simulink model "dual500MHzPFB"  (Simulink 6.2)
settings: Solver=ode45  StartTime=0.0  StopTime=10000  RelTol=1e-3
libraries: xbsIndex_r3 x2070, casper_library x180, xps_library x12, gtkWave x5, gavrt_library x1
(part 15 of 20)

== system dual500MHzPFB/cfgspec/FFT_Subsystem/fft_wideband_real1/fft_biplex_real_4x0/biplex_core/fft_stage_5 ==
  in1 : Inport  Port=1  LatchInput=off
  in2 : Inport  Port=2  LatchInput=off
  of_in : Inport  Port=3  LatchInput=off
  sync : Inport  Port=4  LatchInput=off
  shift : Inport  Port=5  LatchInput=off
  Counter : xbsIndex_r3/Counter  cnt_type=Free Running  n_bits=FFTSize-FFTStage+1  bin_pt=0  arith_type=Unsigned  start_count=0  cnt_to=Inf  cnt_by_val=1  operation=Up  explicit_period=off  period=1  load_pin=off  rst=on  en=off  dbl_ovrd=off  show_param=off  use_rpm=off  gen_core=on
      settings: xl_area=[0, 0, 0, 0, 0, 0, 0]
  Delay : xbsIndex_r3/Delay  latency=1  reg_retiming=off  explicit_period=off  period=1  en=off  accept_only_valid=off  init_zero=on  dbl_ovrd=off  show_param=off
      settings: xl_area=[0, 0, 0, 0, 0, 0, 0]
  Logical1 : xbsIndex_r3/Logical  logical_function=OR  inputs=2  precision=Full  arith_type=Unsigned  n_bits=8  bin_pt=2  align_bp=on  latency=1  explicit_period=on  period=1  en=off  dbl_ovrd=off  show_param=off
      settings: xl_area=[0, 0, 0, 0, 0, 0, 0]
  Mux : xbsIndex_r3/Mux  inputs=2  precision=Full  arith_type="Signed  (2's comp)"  n_bits=8  bin_pt=2  quantization=Truncate  overflow=Wrap  latency=1  explicit_period=off  period=1  en=off  dbl_ovrd=off  show_param=off  mux_type=off  use_rpm=off  gen_core=on
      settings: xl_area=[0, 0, 0, 0, 0, 0, 0]
  Mux1 : xbsIndex_r3/Mux  inputs=2  precision=Full  arith_type="Signed  (2's comp)"  n_bits=8  bin_pt=2  quantization=Truncate  overflow=Wrap  latency=1  explicit_period=off  period=1  en=off  dbl_ovrd=off  show_param=off  mux_type=off  use_rpm=off  gen_core=on
      settings: xl_area=[0, 0, 0, 0, 0, 0, 0]
  Slice : xbsIndex_r3/Slice  Orientation=up  mode=Lower Bit Location + Width  nbits=1  bit1=-(FFTStage - 1)  base1=MSB of Input  bit0=FFTStage - 1  base0=LSB of Input  boolean_output=on  explicit_period=off  period=1  dbl_ovrd=off
  Slice1 : xbsIndex_r3/Slice  mode=Upper Bit Location + Width  nbits=1  bit1=0  base1=MSB of Input  bit0=0  base0=LSB of Input  boolean_output=off  explicit_period=off  period=1  dbl_ovrd=off
  butterfly_direct : Subsystem  AncestorBlock=casper_library/FFTs/butterfly_direct  mask(butterfly_direct){FFTSize=8, Coeffs=[0 1 2 3 4 5 6 7 8 9 10 11 12 13 14 15], StepPeriod=3, BitWidth=18, add_latency=3, mult_latency=3, bram_latency=2, use_bram=0, quantization=Truncate, overflow=Wrap}
      mask prompts: FFTSize "Size of FFT: (2^?)"; Coeffs "Coefficients: (0 to 2^(FFTSize-1)-1)"; StepPeriod "Coefficient Step Period: (2^?)"; BitWidth "Output Bitwidth:"; add_latency "Add Latency"; mult_latency "Mult Latency"; bram_latency "BRAM Latency"; use_bram "Store Coefficients in BRAM"; quantization "Quantization Behavior"; overflow "Overflow Behavior"
      mask init: same as dual500MHzPFB/cfgspec/FFT_Subsystem/fft_wideband_real/fft_direct/butterfly1_0
      settings: AttributesFormatString=|
      | FFTSize=8, Coeffs=[0   1   2   3   4   5   6   7   8   9  10  11  12  13  14  15],
      |  StepPeriod=3, BitWidth=18
      mask StyleString: edit,edit,edit,edit,edit,edit,edit,edit,popup(Truncate|Round  (unbiased: +/- Inf)|Round  (unbiased: Even Values)),popup(Wrap|Saturate|Error)
  delay_b : Subsystem  BlockChoice=delay_slr
      link override delay_bram: bram_latency=bram_latency  DelayLen=2^(FFTSize-FFTStage)
      link override delay_slr: DelayLen=2^(FFTSize-FFTStage)
      settings: AttributesFormatString=%<BlockChoice>  TemplateBlock=casper_library/Delays/delay  MemberBlocks=delay_bram,delay_slr
  delay_f : Subsystem  BlockChoice=delay_slr
      link override delay_bram: bram_latency=bram_latency  DelayLen=2^(FFTSize-FFTStage)
      link override delay_slr: DelayLen=2^(FFTSize-FFTStage)
      settings: AttributesFormatString=%<BlockChoice>  TemplateBlock=casper_library/Delays/delay  MemberBlocks=delay_bram,delay_slr
  sync_delay : casper_library/Delays/sync_delay  DelayLen=2^(FFTSize - FFTStage)
      link override Constant: equ=P=C
      link override Constant1: equ=P=C
      link override Constant2: equ=P=C
      link override Constant3: equ=P=C
  out1 : Outport
  out2 : Outport  Port=2
  of : Outport  Port=3
  sync_out : Outport  Port=4
  wires:
  butterfly_direct/4(sync_out) -> sync_out/1
  butterfly_direct/1(a+bw) -> out1/1
  butterfly_direct/2(a-bw) -> out2/1
  butterfly_direct/3(of) -> Logical1/1
  Slice/1 -> butterfly_direct/4(shift)
  sync_delay/1 -> butterfly_direct/3(sync)
  delay_b/1(Out1) -> butterfly_direct/1(a)
  in2/1 -> delay_f/1(In1)
  Slice1/1 -> Mux1/1, Mux/1
  in1/1 -> Mux1/2, Mux/3
  delay_f/1(Out1) -> Mux/2, Mux1/3
  Mux1/1 -> delay_b/1(In1)
  Mux/1 -> butterfly_direct/2(b)
  Counter/1 -> Slice1/1
  sync/1 -> Delay/1, Counter/1
  Delay/1 -> sync_delay/1
  Logical1/1 -> of/1
  of_in/1 -> Logical1/2
  shift/1 -> Slice/1

== system dual500MHzPFB/cfgspec/FFT_Subsystem/fft_wideband_real1/fft_biplex_real_4x0/biplex_core/fft_stage_6 ==
  in1 : Inport  Port=1  LatchInput=off
  in2 : Inport  Port=2  LatchInput=off
  of_in : Inport  Port=3  LatchInput=off
  sync : Inport  Port=4  LatchInput=off
  shift : Inport  Port=5  LatchInput=off
  Counter : xbsIndex_r3/Counter  cnt_type=Free Running  n_bits=FFTSize-FFTStage+1  bin_pt=0  arith_type=Unsigned  start_count=0  cnt_to=Inf  cnt_by_val=1  operation=Up  explicit_period=off  period=1  load_pin=off  rst=on  en=off  dbl_ovrd=off  show_param=off  use_rpm=off  gen_core=on
      settings: xl_area=[0, 0, 0, 0, 0, 0, 0]
  Delay : xbsIndex_r3/Delay  latency=1  reg_retiming=off  explicit_period=off  period=1  en=off  accept_only_valid=off  init_zero=on  dbl_ovrd=off  show_param=off
      settings: xl_area=[0, 0, 0, 0, 0, 0, 0]
  Logical1 : xbsIndex_r3/Logical  logical_function=OR  inputs=2  precision=Full  arith_type=Unsigned  n_bits=8  bin_pt=2  align_bp=on  latency=1  explicit_period=on  period=1  en=off  dbl_ovrd=off  show_param=off
      settings: xl_area=[0, 0, 0, 0, 0, 0, 0]
  Mux : xbsIndex_r3/Mux  inputs=2  precision=Full  arith_type="Signed  (2's comp)"  n_bits=8  bin_pt=2  quantization=Truncate  overflow=Wrap  latency=1  explicit_period=off  period=1  en=off  dbl_ovrd=off  show_param=off  mux_type=off  use_rpm=off  gen_core=on
      settings: xl_area=[0, 0, 0, 0, 0, 0, 0]
  Mux1 : xbsIndex_r3/Mux  inputs=2  precision=Full  arith_type="Signed  (2's comp)"  n_bits=8  bin_pt=2  quantization=Truncate  overflow=Wrap  latency=1  explicit_period=off  period=1  en=off  dbl_ovrd=off  show_param=off  mux_type=off  use_rpm=off  gen_core=on
      settings: xl_area=[0, 0, 0, 0, 0, 0, 0]
  Slice : xbsIndex_r3/Slice  Orientation=up  mode=Lower Bit Location + Width  nbits=1  bit1=-(FFTStage - 1)  base1=MSB of Input  bit0=FFTStage - 1  base0=LSB of Input  boolean_output=on  explicit_period=off  period=1  dbl_ovrd=off
  Slice1 : xbsIndex_r3/Slice  mode=Upper Bit Location + Width  nbits=1  bit1=0  base1=MSB of Input  bit0=0  base0=LSB of Input  boolean_output=off  explicit_period=off  period=1  dbl_ovrd=off
  butterfly_direct : Subsystem  AncestorBlock=casper_library/FFTs/butterfly_direct  mask(butterfly_direct){FFTSize=8, Coeffs=[0 1 2 3 4 5 6 7 8 9 10 11 12 13 14 15 16 17 18 19 20 21 22 23 24 25 26 27 28 29 30 31], StepPeriod=2, BitWidth=18, add_latency=3, mult_latency=3, bram_latency=2, use_bram=0, quantization=Truncate, overflow=Wrap}
      mask prompts: FFTSize "Size of FFT: (2^?)"; Coeffs "Coefficients: (0 to 2^(FFTSize-1)-1)"; StepPeriod "Coefficient Step Period: (2^?)"; BitWidth "Output Bitwidth:"; add_latency "Add Latency"; mult_latency "Mult Latency"; bram_latency "BRAM Latency"; use_bram "Store Coefficients in BRAM"; quantization "Quantization Behavior"; overflow "Overflow Behavior"
      mask init: same as dual500MHzPFB/cfgspec/FFT_Subsystem/fft_wideband_real/fft_direct/butterfly1_0
      settings: AttributesFormatString=|
      | FFTSize=8, Coeffs=[0   1   2   3   4   5   6   7   8   9  10  11  12  13  14  15  16  17  18  19  20  21  22  23  24  25  26  27  28  29  30  31],
      |  StepPeriod=2, BitWidth=18
      mask StyleString: edit,edit,edit,edit,edit,edit,edit,edit,popup(Truncate|Round  (unbiased: +/- Inf)|Round  (unbiased: Even Values)),popup(Wrap|Saturate|Error)
  delay_b : Subsystem  BlockChoice=delay_slr
      link override delay_bram: bram_latency=bram_latency  DelayLen=2^(FFTSize-FFTStage)
      link override delay_slr: DelayLen=2^(FFTSize-FFTStage)
      settings: AttributesFormatString=%<BlockChoice>  TemplateBlock=casper_library/Delays/delay  MemberBlocks=delay_bram,delay_slr
  delay_f : Subsystem  BlockChoice=delay_slr
      link override delay_bram: bram_latency=bram_latency  DelayLen=2^(FFTSize-FFTStage)
      link override delay_slr: DelayLen=2^(FFTSize-FFTStage)
      settings: AttributesFormatString=%<BlockChoice>  TemplateBlock=casper_library/Delays/delay  MemberBlocks=delay_bram,delay_slr
  sync_delay : casper_library/Delays/sync_delay  DelayLen=2^(FFTSize - FFTStage)
      link override Constant: equ=P=C
      link override Constant1: equ=P=C
      link override Constant2: equ=P=C
      link override Constant3: equ=P=C
  out1 : Outport
  out2 : Outport  Port=2
  of : Outport  Port=3
  sync_out : Outport  Port=4
  wires:
  butterfly_direct/4(sync_out) -> sync_out/1
  butterfly_direct/1(a+bw) -> out1/1
  butterfly_direct/2(a-bw) -> out2/1
  butterfly_direct/3(of) -> Logical1/1
  Slice/1 -> butterfly_direct/4(shift)
  sync_delay/1 -> butterfly_direct/3(sync)
  delay_b/1(Out1) -> butterfly_direct/1(a)
  in2/1 -> delay_f/1(In1)
  Slice1/1 -> Mux1/1, Mux/1
  in1/1 -> Mux1/2, Mux/3
  delay_f/1(Out1) -> Mux/2, Mux1/3
  Mux1/1 -> delay_b/1(In1)
  Mux/1 -> butterfly_direct/2(b)
  Counter/1 -> Slice1/1
  sync/1 -> Delay/1, Counter/1
  Delay/1 -> sync_delay/1
  Logical1/1 -> of/1
  of_in/1 -> Logical1/2
  shift/1 -> Slice/1

== system dual500MHzPFB/cfgspec/FFT_Subsystem/fft_wideband_real1/fft_biplex_real_4x0/biplex_core/fft_stage_7 ==
  in1 : Inport  Port=1  LatchInput=off
  in2 : Inport  Port=2  LatchInput=off
  of_in : Inport  Port=3  LatchInput=off
  sync : Inport  Port=4  LatchInput=off
  shift : Inport  Port=5  LatchInput=off
  Counter : xbsIndex_r3/Counter  cnt_type=Free Running  n_bits=FFTSize-FFTStage+1  bin_pt=0  arith_type=Unsigned  start_count=0  cnt_to=Inf  cnt_by_val=1  operation=Up  explicit_period=off  period=1  load_pin=off  rst=on  en=off  dbl_ovrd=off  show_param=off  use_rpm=off  gen_core=on
      settings: xl_area=[0, 0, 0, 0, 0, 0, 0]
  Delay : xbsIndex_r3/Delay  latency=1  reg_retiming=off  explicit_period=off  period=1  en=off  accept_only_valid=off  init_zero=on  dbl_ovrd=off  show_param=off
      settings: xl_area=[0, 0, 0, 0, 0, 0, 0]
  Logical1 : xbsIndex_r3/Logical  logical_function=OR  inputs=2  precision=Full  arith_type=Unsigned  n_bits=8  bin_pt=2  align_bp=on  latency=1  explicit_period=on  period=1  en=off  dbl_ovrd=off  show_param=off
      settings: xl_area=[0, 0, 0, 0, 0, 0, 0]
  Mux : xbsIndex_r3/Mux  inputs=2  precision=Full  arith_type="Signed  (2's comp)"  n_bits=8  bin_pt=2  quantization=Truncate  overflow=Wrap  latency=1  explicit_period=off  period=1  en=off  dbl_ovrd=off  show_param=off  mux_type=off  use_rpm=off  gen_core=on
      settings: xl_area=[0, 0, 0, 0, 0, 0, 0]
  Mux1 : xbsIndex_r3/Mux  inputs=2  precision=Full  arith_type="Signed  (2's comp)"  n_bits=8  bin_pt=2  quantization=Truncate  overflow=Wrap  latency=1  explicit_period=off  period=1  en=off  dbl_ovrd=off  show_param=off  mux_type=off  use_rpm=off  gen_core=on
      settings: xl_area=[0, 0, 0, 0, 0, 0, 0]
  Slice : xbsIndex_r3/Slice  Orientation=up  mode=Lower Bit Location + Width  nbits=1  bit1=-(FFTStage - 1)  base1=MSB of Input  bit0=FFTStage - 1  base0=LSB of Input  boolean_output=on  explicit_period=off  period=1  dbl_ovrd=off
  Slice1 : xbsIndex_r3/Slice  mode=Upper Bit Location + Width  nbits=1  bit1=0  base1=MSB of Input  bit0=0  base0=LSB of Input  boolean_output=off  explicit_period=off  period=1  dbl_ovrd=off
  butterfly_direct : Subsystem  AncestorBlock=casper_library/FFTs/butterfly_direct  mask(butterfly_direct){FFTSize=8, Coeffs=[0 1 2 3 4 5 6 7 8 9 10 11 12 13 14 15 16 17 18 19 20 21 22 23 24 25 26 27 28 29 30 31 32 33 34 35 36 37 38 39 40 41 42 43 44 45 46 47 48 49 50 51 52 53 54 55 56 57 58 59 60 61 62 63], StepPeriod=1, BitWidth=18, add_latency=3, mult_latency=3, bram_latency=2, use_bram=0, quantization=Truncate, overflow=Wrap}
      mask prompts: FFTSize "Size of FFT: (2^?)"; Coeffs "Coefficients: (0 to 2^(FFTSize-1)-1)"; StepPeriod "Coefficient Step Period: (2^?)"; BitWidth "Output Bitwidth:"; add_latency "Add Latency"; mult_latency "Mult Latency"; bram_latency "BRAM Latency"; use_bram "Store Coefficients in BRAM"; quantization "Quantization Behavior"; overflow "Overflow Behavior"
      mask init: same as dual500MHzPFB/cfgspec/FFT_Subsystem/fft_wideband_real/fft_direct/butterfly1_0
      settings: AttributesFormatString=|
      | FFTSize=8, Coeffs=[0   1   2   3   4   5   6   7   8   9  10  11  12  13  14  15  16  17  18  19  20  21  22  23  24  25  26  27  28  29  30  31  32  33  34  35  36  37  38  39  40  41  42  43  44  45  46  47  48  49  50  51  52  53  54  55  56  57  58  59  60  61  62  63],
      |  StepPeriod=1, BitWidth=18
      mask StyleString: edit,edit,edit,edit,edit,edit,edit,edit,popup(Truncate|Round  (unbiased: +/- Inf)|Round  (unbiased: Even Values)),popup(Wrap|Saturate|Error)
  delay_b : Subsystem  BlockChoice=delay_slr
      link override delay_bram: bram_latency=bram_latency  DelayLen=2^(FFTSize-FFTStage)
      link override delay_slr: DelayLen=2^(FFTSize-FFTStage)
      settings: AttributesFormatString=%<BlockChoice>  TemplateBlock=casper_library/Delays/delay  MemberBlocks=delay_bram,delay_slr
  delay_f : Subsystem  BlockChoice=delay_slr
      link override delay_bram: bram_latency=bram_latency  DelayLen=2^(FFTSize-FFTStage)
      link override delay_slr: DelayLen=2^(FFTSize-FFTStage)
      settings: AttributesFormatString=%<BlockChoice>  TemplateBlock=casper_library/Delays/delay  MemberBlocks=delay_bram,delay_slr
  sync_delay : casper_library/Delays/sync_delay  DelayLen=2^(FFTSize - FFTStage)
      link override Constant: equ=P=C
      link override Constant1: equ=P=C
      link override Constant2: equ=P=C
      link override Constant3: equ=P=C
  out1 : Outport
  out2 : Outport  Port=2
  of : Outport  Port=3
  sync_out : Outport  Port=4
  wires:
  butterfly_direct/4(sync_out) -> sync_out/1
  butterfly_direct/1(a+bw) -> out1/1
  butterfly_direct/2(a-bw) -> out2/1
  butterfly_direct/3(of) -> Logical1/1
  Slice/1 -> butterfly_direct/4(shift)
  sync_delay/1 -> butterfly_direct/3(sync)
  delay_b/1(Out1) -> butterfly_direct/1(a)
  in2/1 -> delay_f/1(In1)
  Slice1/1 -> Mux1/1, Mux/1
  in1/1 -> Mux1/2, Mux/3
  delay_f/1(Out1) -> Mux/2, Mux1/3
  Mux1/1 -> delay_b/1(In1)
  Mux/1 -> butterfly_direct/2(b)
  Counter/1 -> Slice1/1
  sync/1 -> Delay/1, Counter/1
  Delay/1 -> sync_delay/1
  Logical1/1 -> of/1
  of_in/1 -> Logical1/2
  shift/1 -> Slice/1

== system dual500MHzPFB/cfgspec/FFT_Subsystem/fft_wideband_real1/fft_biplex_real_4x0/biplex_core/fft_stage_8 ==
  in1 : Inport  Port=1  LatchInput=off
  in2 : Inport  Port=2  LatchInput=off
  of_in : Inport  Port=3  LatchInput=off
  sync : Inport  Port=4  LatchInput=off
  shift : Inport  Port=5  LatchInput=off
  Counter : xbsIndex_r3/Counter  cnt_type=Free Running  n_bits=FFTSize-FFTStage+1  bin_pt=0  arith_type=Unsigned  start_count=0  cnt_to=Inf  cnt_by_val=1  operation=Up  explicit_period=off  period=1  load_pin=off  rst=on  en=off  dbl_ovrd=off  show_param=off  use_rpm=off  gen_core=on
      settings: xl_area=[0, 0, 0, 0, 0, 0, 0]
  Delay : xbsIndex_r3/Delay  latency=1  reg_retiming=off  explicit_period=off  period=1  en=off  accept_only_valid=off  init_zero=on  dbl_ovrd=off  show_param=off
      settings: xl_area=[0, 0, 0, 0, 0, 0, 0]
  Logical1 : xbsIndex_r3/Logical  logical_function=OR  inputs=2  precision=Full  arith_type=Unsigned  n_bits=8  bin_pt=2  align_bp=on  latency=1  explicit_period=on  period=1  en=off  dbl_ovrd=off  show_param=off
      settings: xl_area=[0, 0, 0, 0, 0, 0, 0]
  Mux : xbsIndex_r3/Mux  inputs=2  precision=Full  arith_type="Signed  (2's comp)"  n_bits=8  bin_pt=2  quantization=Truncate  overflow=Wrap  latency=1  explicit_period=off  period=1  en=off  dbl_ovrd=off  show_param=off  mux_type=off  use_rpm=off  gen_core=on
      settings: xl_area=[0, 0, 0, 0, 0, 0, 0]
  Mux1 : xbsIndex_r3/Mux  inputs=2  precision=Full  arith_type="Signed  (2's comp)"  n_bits=8  bin_pt=2  quantization=Truncate  overflow=Wrap  latency=1  explicit_period=off  period=1  en=off  dbl_ovrd=off  show_param=off  mux_type=off  use_rpm=off  gen_core=on
      settings: xl_area=[0, 0, 0, 0, 0, 0, 0]
  Slice : xbsIndex_r3/Slice  Orientation=up  mode=Lower Bit Location + Width  nbits=1  bit1=-(FFTStage - 1)  base1=MSB of Input  bit0=FFTStage - 1  base0=LSB of Input  boolean_output=on  explicit_period=off  period=1  dbl_ovrd=off
  Slice1 : xbsIndex_r3/Slice  mode=Upper Bit Location + Width  nbits=1  bit1=0  base1=MSB of Input  bit0=0  base0=LSB of Input  boolean_output=off  explicit_period=off  period=1  dbl_ovrd=off
  butterfly_direct : Subsystem  AncestorBlock=casper_library/FFTs/butterfly_direct  mask(butterfly_direct){FFTSize=8, Coeffs=[0 1 2 3 4 5 6 7 8 9 10 11 12 13 14 15 16 17 18 19 20 21 22 23 24 25 26 27 28 29 30 31 32 33 34 35 36 37 38 39 40 41 42 43 44 45 46 47 48 49 50 51 52 53 54 55 56 57 58 59 60 61 62 63 64 65 66 67 68 69 70 71 72 73 74 75 76 77 78 79 80 81 82 83 84 85 86 87 88 89 90 91 92 93 94 95 96 97 98 99 100 101 102 103 104 105 106 107 108 109 110 111 112 113 114 115 116 117 118 119 120 121 122 123 124 125 126 127], StepPeriod=0, BitWidth=18, add_latency=3, mult_latency=3, bram_latency=2, use_bram=0, quantization=Truncate, overflow=Wrap}
      mask prompts: FFTSize "Size of FFT: (2^?)"; Coeffs "Coefficients: (0 to 2^(FFTSize-1)-1)"; StepPeriod "Coefficient Step Period: (2^?)"; BitWidth "Output Bitwidth:"; add_latency "Add Latency"; mult_latency "Mult Latency"; bram_latency "BRAM Latency"; use_bram "Store Coefficients in BRAM"; quantization "Quantization Behavior"; overflow "Overflow Behavior"
      mask init: same as dual500MHzPFB/cfgspec/FFT_Subsystem/fft_wideband_real/fft_direct/butterfly1_0
      settings: AttributesFormatString=|
      | FFTSize=8, Coeffs=[0    1    2    3    4    5    6    7    8    9   10   11   12   13   14   15   16   17   18   19   20   21   22   23   24   25   26   27   28   29   30   31   32   33   34   35   36   37   38   39   40   41   42   43   44   45   46   47   48   49   50   51   52   53   54   55   56   57   58   59   60   61   62   63   64   65   66   67   68   69   70   71   72   73   74   75   76   77   78   79   80   81   82   83   84   85   86   87   88   89   90   91   92   93   94   95   96   97   98   99  100  101  102  103  104  105  106  107  108  109  110  111  112  113  114  115  116  117  118  119  120  121  122  123  124  125  126  127],
      |  StepPeriod=0, BitWidth=18
      mask StyleString: edit,edit,edit,edit,edit,edit,edit,edit,popup(Truncate|Round  (unbiased: +/- Inf)|Round  (unbiased: Even Values)),popup(Wrap|Saturate|Error)
  delay_b : Subsystem  BlockChoice=delay_slr
      link override delay_bram: bram_latency=bram_latency  DelayLen=2^(FFTSize-FFTStage)
      link override delay_slr: DelayLen=2^(FFTSize-FFTStage)
      settings: AttributesFormatString=%<BlockChoice>  TemplateBlock=casper_library/Delays/delay  MemberBlocks=delay_bram,delay_slr
  delay_f : Subsystem  BlockChoice=delay_slr
      link override delay_bram: bram_latency=bram_latency  DelayLen=2^(FFTSize-FFTStage)
      link override delay_slr: DelayLen=2^(FFTSize-FFTStage)
      settings: AttributesFormatString=%<BlockChoice>  TemplateBlock=casper_library/Delays/delay  MemberBlocks=delay_bram,delay_slr
  sync_delay : casper_library/Delays/sync_delay  DelayLen=2^(FFTSize - FFTStage)
      link override Constant: equ=P=C
      link override Constant1: equ=P=C
      link override Constant2: equ=P=C
      link override Constant3: equ=P=C
  out1 : Outport
  out2 : Outport  Port=2
  of : Outport  Port=3
  sync_out : Outport  Port=4
  wires:
  butterfly_direct/4(sync_out) -> sync_out/1
  butterfly_direct/1(a+bw) -> out1/1
  butterfly_direct/2(a-bw) -> out2/1
  butterfly_direct/3(of) -> Logical1/1
  Slice/1 -> butterfly_direct/4(shift)
  sync_delay/1 -> butterfly_direct/3(sync)
  delay_b/1(Out1) -> butterfly_direct/1(a)
  in2/1 -> delay_f/1(In1)
  Slice1/1 -> Mux1/1, Mux/1
  in1/1 -> Mux1/2, Mux/3
  delay_f/1(Out1) -> Mux/2, Mux1/3
  Mux1/1 -> delay_b/1(In1)
  Mux/1 -> butterfly_direct/2(b)
  Counter/1 -> Slice1/1
  sync/1 -> Delay/1, Counter/1
  Delay/1 -> sync_delay/1
  Logical1/1 -> of/1
  of_in/1 -> Logical1/2
  shift/1 -> Slice/1

== system dual500MHzPFB/cfgspec/FFT_Subsystem/fft_wideband_real1/fft_direct/butterfly1_0/twiddle ==
  a : Inport  Port=1  LatchInput=off
  b : Inport  Port=2  LatchInput=off
  sync : Inport  Port=3  LatchInput=off
  twiddle_general_3mult : casper_library/FFTs/Twiddle/twiddle_general_3mult  Coeffs="[1+0i               0.99992-0.012272i         0.9997-0.024541i        0.99932-0.036807i         0.9988-0.049068i        0.99812-0.061321i        0.99729-0.073565i        0.99631-0.085797i        0.99518-0.098017i        0.99391-0.11022i         0.99248-0.12241i          0.9909-0.13458i         0.98918-0.14673i          0.9873-0.15886i         0.98528-0.17096i         0.98311-0.18304i         0.98079-0.19509i         0.97832-0.20711i          0.9757-0.2191i          0.97294-0.23106i         0.97003-0.24298i         0.96698-0.25487i         0.96378-0.26671i         0.96043-0.27852i         0.95694-0.29028i         0.95331-0.30201i         0.94953-0.31368i         0.94561-0.32531i         0.94154-0.33689i         0.93734-0.34842i         0.93299-0.3599i          0.92851-0.37132i         0.92388-0.38268i         0.91911-0.39399i         0.91421-0.40524i         0.90917-0.41643i         0.90399-0.42756i         0.89867-0.43862i         0.89322-0.44961i         0.88764-0.46054i         0.88192-0.4714i          0.87607-0.48218i         0.87009-0.4929i          0.86397-0.50354i         0.85773-0.5141i          0.85136-0.52459i         0.84485-0.535i           0.83822-0.54532i         0.83147-0.55557i         0.82459-0.56573i         0.81758-0.57581i         0.81046-0.5858i          0.80321-0.5957i          0.79584-0.60551i         0.78835-0.61523i         0.78074-0.62486i         0.77301-0.63439i         0.76517-0.64383i         0.75721-0.65317i         0.74914-0.66242i         0.74095-0.67156i         0.73265-0.6806i          0.72425-0.68954i         0.71573-0.69838i         0.70711-0.70711i         0.69838-0.71573i         0.68954-0.72425i          0.6806-0.73265i         0.67156-0.74095i         0.66242-0.74914i         0.65317-0.75721i         0.64383-0.76517i         0.63439-0.77301i         0.62486-0.78074i         0.61523-0.78835i         0.60551-0.79584i          0.5957-0.80321i          0.5858-0.81046i         0.57581-0.81758i         0.56573-0.82459i         0.55557-0.83147i         0.54532-0.83822i           0.535-0.84485i         0.52459-0.85136i          0.5141-0.85773i         0.50354-0.86397i          0.4929-0.87009i         0.48218-0.87607i          0.4714-0.88192i         0.46054-0.88764i         0.44961-0.89322i         0.43862-0.89867i         0.42756-0.90399i         0.41643-0.90917i         0.40524-0.91421i         0.39399-0.91911i         0.38268-0.92388i         0.37132-0.92851i          0.3599-0.93299i         0.34842-0.93734i         0.33689-0.94154i         0.32531-0.94561i         0.31368-0.94953i         0.30201-0.95331i         0.29028-0.95694i         0.27852-0.96043i         0.26671-0.96378i         0.25487-0.96698i         0.24298-0.97003i         0.23106-0.97294i          0.2191-0.9757i          0.20711-0.97832i         0.19509-0.98079i         0.18304-0.98311i         0.17096-0.98528i         0.15886-0.9873i          0.14673-0.98918i         0.13458-0.9909i          0.12241-0.99248i         0.11022-0.99391i        0.098017-0.99518i        0.085797-0.99631i        0.073565-0.99729i        0.061321-0.99812i        0.049068-0.9988i         0.036807-0.99932i        0.024541-0.9997i         0.012272-0.99992i     6.1232e-017-1i             -0.012272-0.99992i       -0.024541-0.9997i        -0.036807-0.99932i       -0.049068-0.9988i        -0.061321-0.99812i       -0.073565-0.99729i       -0.085797-0.99631i       -0.098017-0.99518i        -0.11022-0.99391i        -0.12241-0.99248i        -0.13458-0.9909i         -0.14673-0.98918i        -0.15886-0.9873i         -0.17096-0.98528i        -0.18304-0.98311i        -0.19509-0.98079i        -0.20711-0.97832i         -0.2191-0.9757i         -0.23106-0.97294i        -0.24298-0.97003i        -0.25487-0.96698i        -0.26671-0.96378i        -0.27852-0.96043i        -0.29028-0.95694i        -0.30201-0.95331i        -0.31368-0.94953i        -0.32531-0.94561i        -0.33689-0.94154i        -0.34842-0.93734i         -0.3599-0.93299i        -0.37132-0.92851i ...(+2394 chars)   ]"  StepPeriod=0  BitWidth=18  add_latency=3  mult_latency=3  bram_latency=2
  a_re : Outport
  a_im : Outport  Port=2
  bw_re : Outport  Port=3
  bw_im : Outport  Port=4
  sync_out : Outport  Port=5
  wires:
  a/1 -> twiddle_general_3mult/1
  b/1 -> twiddle_general_3mult/2
  sync/1 -> twiddle_general_3mult/3
  twiddle_general_3mult/1 -> a_re/1
  twiddle_general_3mult/2 -> a_im/1
  twiddle_general_3mult/3 -> bw_re/1
  twiddle_general_3mult/4 -> bw_im/1
  twiddle_general_3mult/5 -> sync_out/1

== system dual500MHzPFB/cfgspec/FFT_Subsystem/fft_wideband_real1/fft_direct/butterfly1_1/twiddle ==
  a : Inport  Port=1  LatchInput=off
  b : Inport  Port=2  LatchInput=off
  sync : Inport  Port=3  LatchInput=off
  twiddle_general_3mult : casper_library/FFTs/Twiddle/twiddle_general_3mult  Coeffs="[1+0i               0.99992-0.012272i         0.9997-0.024541i        0.99932-0.036807i         0.9988-0.049068i        0.99812-0.061321i        0.99729-0.073565i        0.99631-0.085797i        0.99518-0.098017i        0.99391-0.11022i         0.99248-0.12241i          0.9909-0.13458i         0.98918-0.14673i          0.9873-0.15886i         0.98528-0.17096i         0.98311-0.18304i         0.98079-0.19509i         0.97832-0.20711i          0.9757-0.2191i          0.97294-0.23106i         0.97003-0.24298i         0.96698-0.25487i         0.96378-0.26671i         0.96043-0.27852i         0.95694-0.29028i         0.95331-0.30201i         0.94953-0.31368i         0.94561-0.32531i         0.94154-0.33689i         0.93734-0.34842i         0.93299-0.3599i          0.92851-0.37132i         0.92388-0.38268i         0.91911-0.39399i         0.91421-0.40524i         0.90917-0.41643i         0.90399-0.42756i         0.89867-0.43862i         0.89322-0.44961i         0.88764-0.46054i         0.88192-0.4714i          0.87607-0.48218i         0.87009-0.4929i          0.86397-0.50354i         0.85773-0.5141i          0.85136-0.52459i         0.84485-0.535i           0.83822-0.54532i         0.83147-0.55557i         0.82459-0.56573i         0.81758-0.57581i         0.81046-0.5858i          0.80321-0.5957i          0.79584-0.60551i         0.78835-0.61523i         0.78074-0.62486i         0.77301-0.63439i         0.76517-0.64383i         0.75721-0.65317i         0.74914-0.66242i         0.74095-0.67156i         0.73265-0.6806i          0.72425-0.68954i         0.71573-0.69838i         0.70711-0.70711i         0.69838-0.71573i         0.68954-0.72425i          0.6806-0.73265i         0.67156-0.74095i         0.66242-0.74914i         0.65317-0.75721i         0.64383-0.76517i         0.63439-0.77301i         0.62486-0.78074i         0.61523-0.78835i         0.60551-0.79584i          0.5957-0.80321i          0.5858-0.81046i         0.57581-0.81758i         0.56573-0.82459i         0.55557-0.83147i         0.54532-0.83822i           0.535-0.84485i         0.52459-0.85136i          0.5141-0.85773i         0.50354-0.86397i          0.4929-0.87009i         0.48218-0.87607i          0.4714-0.88192i         0.46054-0.88764i         0.44961-0.89322i         0.43862-0.89867i         0.42756-0.90399i         0.41643-0.90917i         0.40524-0.91421i         0.39399-0.91911i         0.38268-0.92388i         0.37132-0.92851i          0.3599-0.93299i         0.34842-0.93734i         0.33689-0.94154i         0.32531-0.94561i         0.31368-0.94953i         0.30201-0.95331i         0.29028-0.95694i         0.27852-0.96043i         0.26671-0.96378i         0.25487-0.96698i         0.24298-0.97003i         0.23106-0.97294i          0.2191-0.9757i          0.20711-0.97832i         0.19509-0.98079i         0.18304-0.98311i         0.17096-0.98528i         0.15886-0.9873i          0.14673-0.98918i         0.13458-0.9909i          0.12241-0.99248i         0.11022-0.99391i        0.098017-0.99518i        0.085797-0.99631i        0.073565-0.99729i        0.061321-0.99812i        0.049068-0.9988i         0.036807-0.99932i        0.024541-0.9997i         0.012272-0.99992i     6.1232e-017-1i             -0.012272-0.99992i       -0.024541-0.9997i        -0.036807-0.99932i       -0.049068-0.9988i        -0.061321-0.99812i       -0.073565-0.99729i       -0.085797-0.99631i       -0.098017-0.99518i        -0.11022-0.99391i        -0.12241-0.99248i        -0.13458-0.9909i         -0.14673-0.98918i        -0.15886-0.9873i         -0.17096-0.98528i        -0.18304-0.98311i        -0.19509-0.98079i        -0.20711-0.97832i         -0.2191-0.9757i         -0.23106-0.97294i        -0.24298-0.97003i        -0.25487-0.96698i        -0.26671-0.96378i        -0.27852-0.96043i        -0.29028-0.95694i        -0.30201-0.95331i        -0.31368-0.94953i        -0.32531-0.94561i        -0.33689-0.94154i        -0.34842-0.93734i         -0.3599-0.93299i        -0.37132-0.92851i ...(+2394 chars)   ]"  StepPeriod=0  BitWidth=18  add_latency=3  mult_latency=3  bram_latency=2
  a_re : Outport
  a_im : Outport  Port=2
  bw_re : Outport  Port=3
  bw_im : Outport  Port=4
  sync_out : Outport  Port=5
  wires:
  a/1 -> twiddle_general_3mult/1
  b/1 -> twiddle_general_3mult/2
  sync/1 -> twiddle_general_3mult/3
  twiddle_general_3mult/1 -> a_re/1
  twiddle_general_3mult/2 -> a_im/1
  twiddle_general_3mult/3 -> bw_re/1
  twiddle_general_3mult/4 -> bw_im/1
  twiddle_general_3mult/5 -> sync_out/1

== system dual500MHzPFB/cfgspec/FFT_Subsystem/fft_wideband_real1/fft_direct/butterfly2_0/twiddle ==
  a : Inport  Port=1  LatchInput=off
  b : Inport  Port=2  LatchInput=off
  sync : Inport  Port=3  LatchInput=off
  twiddle_general_3mult : casper_library/FFTs/Twiddle/twiddle_general_3mult  Coeffs="[1+0i               0.99998-0.0061359i       0.99992-0.012272i        0.99983-0.018407i         0.9997-0.024541i        0.99953-0.030675i        0.99932-0.036807i        0.99908-0.042938i         0.9988-0.049068i        0.99848-0.055195i        0.99812-0.061321i        0.99772-0.067444i        0.99729-0.073565i        0.99682-0.079682i        0.99631-0.085797i        0.99577-0.091909i        0.99518-0.098017i        0.99456-0.10412i         0.99391-0.11022i         0.99321-0.11632i         0.99248-0.12241i         0.99171-0.1285i           0.9909-0.13458i         0.99006-0.14066i         0.98918-0.14673i         0.98826-0.1528i           0.9873-0.15886i         0.98631-0.16491i         0.98528-0.17096i         0.98421-0.177i           0.98311-0.18304i         0.98196-0.18907i         0.98079-0.19509i         0.97957-0.2011i          0.97832-0.20711i         0.97703-0.21311i          0.9757-0.2191i          0.97434-0.22508i         0.97294-0.23106i          0.9715-0.23702i         0.97003-0.24298i         0.96852-0.24893i         0.96698-0.25487i         0.96539-0.26079i         0.96378-0.26671i         0.96212-0.27262i         0.96043-0.27852i          0.9587-0.28441i         0.95694-0.29028i         0.95514-0.29615i         0.95331-0.30201i         0.95144-0.30785i         0.94953-0.31368i         0.94759-0.3195i          0.94561-0.32531i         0.94359-0.33111i         0.94154-0.33689i         0.93946-0.34266i         0.93734-0.34842i         0.93518-0.35416i         0.93299-0.3599i          0.93077-0.36561i         0.92851-0.37132i         0.92621-0.37701i         0.92388-0.38268i         0.92151-0.38835i         0.91911-0.39399i         0.91668-0.39962i         0.91421-0.40524i         0.91171-0.41084i         0.90917-0.41643i          0.9066-0.422i           0.90399-0.42756i         0.90135-0.43309i         0.89867-0.43862i         0.89597-0.44412i         0.89322-0.44961i         0.89045-0.45508i         0.88764-0.46054i          0.8848-0.46598i         0.88192-0.4714i          0.87901-0.4768i          0.87607-0.48218i         0.87309-0.48755i         0.87009-0.4929i          0.86705-0.49823i         0.86397-0.50354i         0.86087-0.50883i         0.85773-0.5141i          0.85456-0.51936i         0.85136-0.52459i         0.84812-0.5298i          0.84485-0.535i           0.84155-0.54017i         0.83822-0.54532i         0.83486-0.55046i         0.83147-0.55557i         0.82805-0.56066i         0.82459-0.56573i          0.8211-0.57078i         0.81758-0.57581i         0.81404-0.58081i         0.81046-0.5858i          0.80685-0.59076i         0.80321-0.5957i          0.79954-0.60062i         0.79584-0.60551i         0.79211-0.61038i         0.78835-0.61523i         0.78456-0.62006i         0.78074-0.62486i         0.77689-0.62964i         0.77301-0.63439i          0.7691-0.63912i         0.76517-0.64383i          0.7612-0.64851i         0.75721-0.65317i         0.75319-0.65781i         0.74914-0.66242i         0.74506-0.667i           0.74095-0.67156i         0.73682-0.67609i         0.73265-0.6806i          0.72846-0.68508i         0.72425-0.68954i            0.72-0.69397i         0.71573-0.69838i         0.71143-0.70275i         0.70711-0.70711i         0.70275-0.71143i         0.69838-0.71573i         0.69397-0.72i            0.68954-0.72425i         0.68508-0.72846i          0.6806-0.73265i         0.67609-0.73682i         0.67156-0.74095i           0.667-0.74506i         0.66242-0.74914i         0.65781-0.75319i         0.65317-0.75721i         0.64851-0.7612i          0.64383-0.76517i         0.63912-0.7691i          0.63439-0.77301i         0.62964-0.77689i         0.62486-0.78074i         0.62006-0.78456i         0.61523-0.78835i         0.61038-0.79211i         0.60551-0.79584i         0.60062-0.79954i          0.5957-0.80321i         0.59076-0.80685i          0.5858-0.81046i         0.58081-0.81404i         0.57581-0.81758i         0.57078-0.8211i          0.56573-0.82459i         0.56066-0.82805i ...(+2392 chars)    ]"  StepPeriod=0  BitWidth=18  add_latency=3  mult_latency=3  bram_latency=2
  a_re : Outport
  a_im : Outport  Port=2
  bw_re : Outport  Port=3
  bw_im : Outport  Port=4
  sync_out : Outport  Port=5
  wires:
  a/1 -> twiddle_general_3mult/1
  b/1 -> twiddle_general_3mult/2
  sync/1 -> twiddle_general_3mult/3
  twiddle_general_3mult/1 -> a_re/1
  twiddle_general_3mult/2 -> a_im/1
  twiddle_general_3mult/3 -> bw_re/1
  twiddle_general_3mult/4 -> bw_im/1
  twiddle_general_3mult/5 -> sync_out/1

== system dual500MHzPFB/cfgspec/FFT_Subsystem/fft_wideband_real1/fft_direct/butterfly2_1/twiddle ==
  a : Inport  Port=1  LatchInput=off
  b : Inport  Port=2  LatchInput=off
  sync : Inport  Port=3  LatchInput=off
  twiddle_general_3mult : casper_library/FFTs/Twiddle/twiddle_general_3mult  Coeffs="[6.1232e-017-1i            -0.0061359-0.99998i       -0.012272-0.99992i       -0.018407-0.99983i       -0.024541-0.9997i        -0.030675-0.99953i       -0.036807-0.99932i       -0.042938-0.99908i       -0.049068-0.9988i        -0.055195-0.99848i       -0.061321-0.99812i       -0.067444-0.99772i       -0.073565-0.99729i       -0.079682-0.99682i       -0.085797-0.99631i       -0.091909-0.99577i       -0.098017-0.99518i        -0.10412-0.99456i        -0.11022-0.99391i        -0.11632-0.99321i        -0.12241-0.99248i         -0.1285-0.99171i        -0.13458-0.9909i         -0.14066-0.99006i        -0.14673-0.98918i         -0.1528-0.98826i        -0.15886-0.9873i         -0.16491-0.98631i        -0.17096-0.98528i          -0.177-0.98421i        -0.18304-0.98311i        -0.18907-0.98196i        -0.19509-0.98079i         -0.2011-0.97957i        -0.20711-0.97832i        -0.21311-0.97703i         -0.2191-0.9757i         -0.22508-0.97434i        -0.23106-0.97294i        -0.23702-0.9715i         -0.24298-0.97003i        -0.24893-0.96852i        -0.25487-0.96698i        -0.26079-0.96539i        -0.26671-0.96378i        -0.27262-0.96212i        -0.27852-0.96043i        -0.28441-0.9587i         -0.29028-0.95694i        -0.29615-0.95514i        -0.30201-0.95331i        -0.30785-0.95144i        -0.31368-0.94953i         -0.3195-0.94759i        -0.32531-0.94561i        -0.33111-0.94359i        -0.33689-0.94154i        -0.34266-0.93946i        -0.34842-0.93734i        -0.35416-0.93518i         -0.3599-0.93299i        -0.36561-0.93077i        -0.37132-0.92851i        -0.37701-0.92621i        -0.38268-0.92388i        -0.38835-0.92151i        -0.39399-0.91911i        -0.39962-0.91668i        -0.40524-0.91421i        -0.41084-0.91171i        -0.41643-0.90917i          -0.422-0.9066i         -0.42756-0.90399i        -0.43309-0.90135i        -0.43862-0.89867i        -0.44412-0.89597i        -0.44961-0.89322i        -0.45508-0.89045i        -0.46054-0.88764i        -0.46598-0.8848i          -0.4714-0.88192i         -0.4768-0.87901i        -0.48218-0.87607i        -0.48755-0.87309i         -0.4929-0.87009i        -0.49823-0.86705i        -0.50354-0.86397i        -0.50883-0.86087i         -0.5141-0.85773i        -0.51936-0.85456i        -0.52459-0.85136i         -0.5298-0.84812i          -0.535-0.84485i        -0.54017-0.84155i        -0.54532-0.83822i        -0.55046-0.83486i        -0.55557-0.83147i        -0.56066-0.82805i        -0.56573-0.82459i        -0.57078-0.8211i         -0.57581-0.81758i        -0.58081-0.81404i         -0.5858-0.81046i        -0.59076-0.80685i         -0.5957-0.80321i        -0.60062-0.79954i        -0.60551-0.79584i        -0.61038-0.79211i        -0.61523-0.78835i        -0.62006-0.78456i        -0.62486-0.78074i        -0.62964-0.77689i        -0.63439-0.77301i        -0.63912-0.7691i         -0.64383-0.76517i        -0.64851-0.7612i         -0.65317-0.75721i        -0.65781-0.75319i        -0.66242-0.74914i          -0.667-0.74506i        -0.67156-0.74095i        -0.67609-0.73682i         -0.6806-0.73265i        -0.68508-0.72846i        -0.68954-0.72425i        -0.69397-0.72i           -0.69838-0.71573i        -0.70275-0.71143i        -0.70711-0.70711i        -0.71143-0.70275i        -0.71573-0.69838i           -0.72-0.69397i        -0.72425-0.68954i        -0.72846-0.68508i        -0.73265-0.6806i         -0.73682-0.67609i        -0.74095-0.67156i        -0.74506-0.667i          -0.74914-0.66242i        -0.75319-0.65781i        -0.75721-0.65317i         -0.7612-0.64851i        -0.76517-0.64383i         -0.7691-0.63912i        -0.77301-0.63439i        -0.77689-0.62964i        -0.78074-0.62486i        -0.78456-0.62006i        -0.78835-0.61523i        -0.79211-0.61038i        -0.79584-0.60551i        -0.79954-0.60062i        -0.80321-0.5957i         -0.80685-0.59076i        -0.81046-0.5858i         -0.81404-0.58081i        -0.81758-0.57581i         -0.8211-0.57078i        -0.82459-0.56573i        -0.82805-0.56066i ...(+2399 chars)  ]"  StepPeriod=0  BitWidth=18  add_latency=3  mult_latency=3  bram_latency=2
  a_re : Outport
  a_im : Outport  Port=2
  bw_re : Outport  Port=3
  bw_im : Outport  Port=4
  sync_out : Outport  Port=5
  wires:
  a/1 -> twiddle_general_3mult/1
  b/1 -> twiddle_general_3mult/2
  sync/1 -> twiddle_general_3mult/3
  twiddle_general_3mult/1 -> a_re/1
  twiddle_general_3mult/2 -> a_im/1
  twiddle_general_3mult/3 -> bw_re/1
  twiddle_general_3mult/4 -> bw_im/1
  twiddle_general_3mult/5 -> sync_out/1
